simulink model "SMC"  (R2022a)
settings: Solver=ode4  StartTime=0.0  StopTime=30  FixedStep=0.0002  RelTol=1e-3  EnableMultiTasking=on
InitFcn:
  | clc
  | clear
  | x=[    1.0000
  |    -1.0000
  |    -1.0000
  |    -1.0000
  |     1.0000
  |     1.0000
  |     1.0000
  |    -1.0000
  |    -1.0000
  |    -0.0461
  |    -0.2275
  |    -1.0000
  |     1.0000
  |     1.0000
  |     1.0000
  |     1.0000
  |     0.1336
  |    -0.0153
  |    -0.9258
  |     1.0000
  |     1.0000
  |     1.0000
  |    -1.0000
  |     1.0000
  |    -1.0000
  |     1.0000];
  | 
  | x=x';
  | 
  | alpha = 20+5*x(1);
  | beta = 4+2*x(2);
  | 
  | gamma2 = 1.2 + 0.3* x(3);
  | gamma1 = 1.2 + 0.3* x(4);
  | 
  | eta1 = 2.5 + 0.5*x(5);
  | eta2 = 0.3 + 0.1*x(6);
  | 
  | 
  | w1 =25* x(7:15);
  | w4 =abs(5* x(16:24));
  | b1 = 2 + x(25);
  | b4 = 2 + x(26);
  | 
  | 
  | center1=[-0.5 0 0.5];
  | center2=[-2 0 2];
  | 
  | sigma1 = [0.2 0.2 0.2];
  | sigma2 = [0.6 0.6 0.6];
  | 
  | x1=[     1.0000
  |    -0.7700
  |    -0.9968
  |    -0.7959
  |    -0.3103
  |    -0.2531
  |     0.7496
  |     0.6290
  |    -0.6185
  |    -0.2913
  |     0.0215
  |    -0.1400
  |     0.0582
  |     0.8560
  |     0.2296
  |    -0.4623
  |     0.4590
  |    -0.3154
  |     0.7435
  |     0.3255
  |     0.1149
  |    -0.2814
  |    -0.4088
  |     0.2365
  |    -0.7489
  |    -0.0827];
  | 
  | alpha_1 = 22+6*x1(1);
  | beta_1 =5+2*x1(2);
  | 
  | gamma2_1 = 1.2 + 0.4* x1(3);
  | gamma1_1 = 1.2 + 0.4* x1(4);
  | 
  | eta1_1 = 2.5 + 0.5*x1(5);
  | eta2_1 = 0.3 + 0.1*x1(6);
  | 
  | S = 0;
  | 
  | w1_1 =30* x1(7:15) + 5;
  | w4_1 =abs(5* x1(16:24));
StopFcn:
  | save('SMC.mat')
settings Model: Creator=Ali.Assareh  LastModifiedBy=MohammadAli
settings SolverCC: AlgebraicLoopSolver=TrustRegion
settings DataIOCC: LimitDataPoints=on  SaveFormat=Array  ReturnWorkspaceOutputs=off
settings OptimizationCC: LifeSpan=inf
settings DebuggingCC: UnderspecifiedInitializationDetection=Classic  MergeDetectMultiDrivingBlocksExec=none  SolverPrmCheckMsg=warning  UnconnectedInputMsg=warning  UnconnectedOutputMsg=warning  UnconnectedLineMsg=warning  StateNameClashWarn=warning  SFUnexpectedBacktrackingDiag=warning  SFNoUnconditionalDefaultTransitionDiag=warning  SFExecutionAtInitializationDiag=none  SFMachineParentedDataDiag=warning  ArithmeticOperatorsInVariantConditions=warning
settings HardwareCC: ProdBitPerPointer=32  ProdBitPerSizeT=32  ProdBitPerPtrDiffT=32  ProdLargestAtomicFloat=None  ProdIntDivRoundTo=Undefined  ProdEndianess=Unspecified  ProdWordSize=32  ProdHWDeviceType=32-bit Generic
settings ModelReferenceCC: PropagateSignalLabelsOutOfModel=off
settings SFSimCC: SimUseLocalCustomCode=off  CustomCodeUndefinedFunction=UseInterfaceOnly
settings RTWCC: RTWUseLocalCustomCode=off  DLArmComputeVersion=19.05
settings CodeAppCC: StateflowObjectComments=on
settings GRTTargetCC: TargetLangStandard=C89/C90 (ANSI)
settings ConfigComp: CovMetricSettings=dw  CovSaveCumulativeToWorkspaceVar=on  CovSaveSingleToWorkspaceVar=on  CovExternalEMLEnable=off

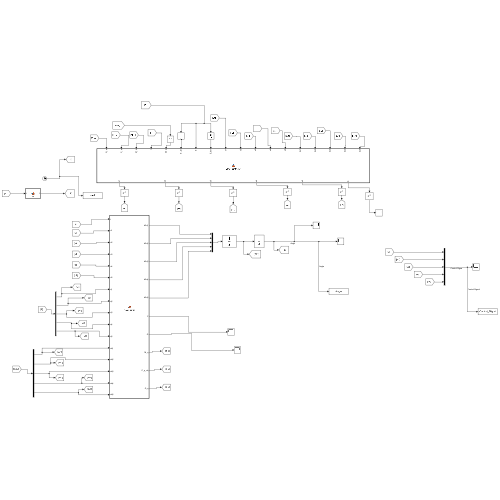
[thumbnail: Simulink's stored preview of the top-level diagram]
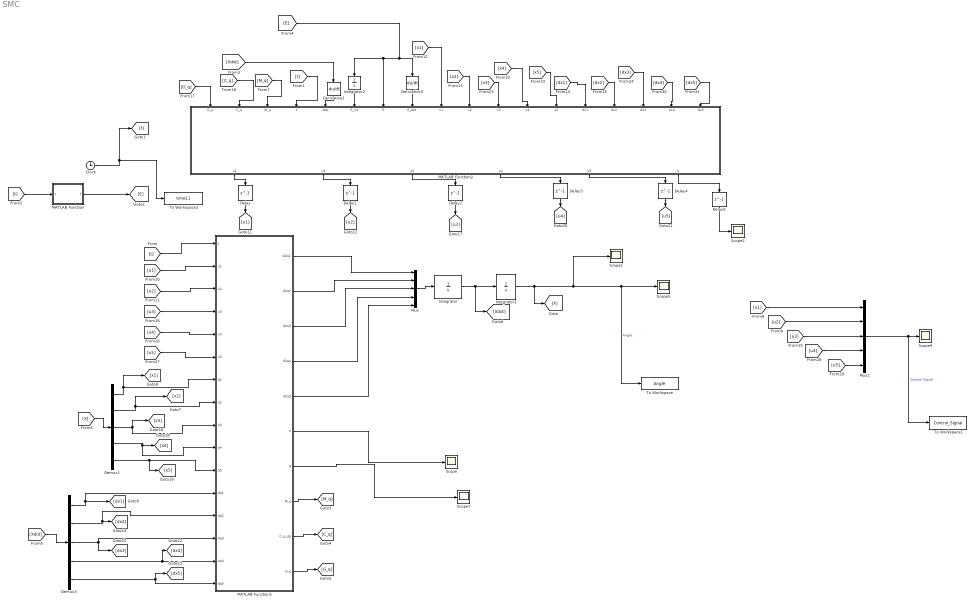
== system SMC ==
  Clock : Clock
  Delay{,1..4,6} (6 alike) : Delay  DelayLength=1  InitialCondition=0
  Demux1 : Demux  Outputs=5
  Demux3 : Demux  Outputs=5
  Derivative1 : Derivative
  Derivative3 : Derivative
  Integrator : Integrator  InitialCondition=[0.4;-0.8;1;0.3;0.1]*1
  Integrator1 : Integrator  InitialCondition=[-0.4;0.8;0.4;-1.7;1.1]*1
  Integrator2 : Integrator
  MATLAB Function : MATLAB Function  TreatAsAtomicUnit=on
  MATLAB Function1 : MATLAB Function  TreatAsAtomicUnit=on
  MATLAB Function2 : MATLAB Function  TreatAsAtomicUnit=on
  Mux : Mux  Inputs=5
  Mux1 : Mux  Inputs=5
  Scope{,1..2,5,7,9} (6 alike) : Scope
  To Workspace : ToWorkspace  VariableName=Angle  SampleTime=-1
  To Workspace1 : ToWorkspace  VariableName=Control_Signal  SampleTime=-1
  To Workspace2 : ToWorkspace  VariableName=time11  SampleTime=-1
  wires:
  MATLAB Function1/1(d2q1) -> Mux/1
  MATLAB Function1/2(d2q2) -> Mux/2
  Integrator/1 -> [Xdot], Integrator1/1
  Mux/1 -> Integrator/1
  Demux3/2 -> MATLAB Function1/13(dq2), [dx2]
  Demux3/1 -> MATLAB Function1/12(dq1), [dx1]
  Clock/1 -> [t], To Workspace2/1
  MATLAB Function2/2(u2) -> Delay1/1
  [t] -> MATLAB Function1/1(t)
  [t] -> MATLAB Function2/4(t)
  [Xdot] -> Demux3/1
  [X] -> Demux1/1
  [E] -> MATLAB Function2/7(E), Integrator2/1, Derivative3/1
  Demux1/1 -> [x1], MATLAB Function1/7(q1)
  Demux1/2 -> MATLAB Function1/8(q2), [x2]
  MATLAB Function2/1(u1) -> Delay/1
  [u1] -> MATLAB Function1/2(u1)
  [u2] -> MATLAB Function1/3(u2)
  MATLAB Function1/7(G) -> Scope7/1
  MATLAB Function1/6(F) -> Scope/1
  Derivative3/1 -> MATLAB Function2/8(E_dot)
  [x1] -> MATLAB Function2/9(x1)
  [x2] -> MATLAB Function2/10(x2)
  [u1] -> Mux1/1
  [u2] -> Mux1/2
  MATLAB Function1/3(d2q3) -> Mux/3
  [u3] -> MATLAB Function1/4(u3)
  Demux3/3 -> MATLAB Function1/14(dq3), [dx3]
  Demux1/3 -> [x3], MATLAB Function1/9(q3)
  MATLAB Function2/3(u3) -> Delay2/1
  [u3] -> Mux1/3
  [x3] -> MATLAB Function2/11(x3)
  [dx3] -> MATLAB Function2/16(dx3)
  MATLAB Function1/4(d2q4) -> Mux/4
  MATLAB Function1/5(d2q5) -> Mux/5
  [u4] -> MATLAB Function1/5(u4)
  [u5] -> MATLAB Function1/6(u5)
  Demux1/4 -> MATLAB Function1/10(q4), [x4]
  Demux1/5 -> MATLAB Function1/11(q5), [x5]
  MATLAB Function2/5(u5) -> Delay4/1
  MATLAB Function2/4(u4) -> Delay3/1
  [u4] -> Mux1/4
  [u5] -> Mux1/5
  Demux3/4 -> [dx4], MATLAB Function1/15(dq4)
  Demux3/5 -> [dx5], MATLAB Function1/16(dq5)
  [dx5] -> MATLAB Function2/18(dx5)
  [x4] -> MATLAB Function2/12(x4)
  [x5] -> MATLAB Function2/13(x5)
  [dx1] -> MATLAB Function2/14(dx1)
  [dx2] -> MATLAB Function2/15(dx2)
  [dx4] -> MATLAB Function2/17(dx4)
  [t] -> MATLAB Function/1(t)
  MATLAB Function/1(f) -> [E]
  Integrator2/1 -> MATLAB Function2/6(E_int)
  [Xdot] -> Derivative1/1
  Derivative1/1 -> MATLAB Function2/5(ddq)
  MATLAB Function1/8(M_q) -> [M_q]
  MATLAB Function1/9(C_q_dq) -> [C_q]
  MATLAB Function1/10(G_q) -> [G_q]
  [M_q] -> MATLAB Function2/3(M_q)
  [C_q] -> MATLAB Function2/2(C_q)
  [G_q] -> MATLAB Function2/1(G_q)
  Delay/1 -> [u1]
  Delay1/1 -> [u2]
  Delay2/1 -> [u3]
  Delay3/1 -> [u4]
  Delay4/1 -> [u5]
  Integrator1/1 -> Scope1/1, To Workspace/1, Scope5/1, [X]  "Angle"
  Mux1/1 -> To Workspace1/1, Scope9/1  "Control Signal"
  MATLAB Function2/6(S) -> Delay6/1
  Delay6/1 -> Scope2/1

== matlab function SMC/MATLAB Function1 ==
  data: t input; u1 input; d2q1 output; u2 input; u3 input; u4 input; u5 input; q1 input; q2 input; q3 input; q4 input; q5 input; dq1 input; dq2 input; d2q2 output; d2q3 output; d2q4 output; d2q5 output; F output; G output; dq3 input; dq4 input; dq5 input; M_q output; C_q_dq output; G_q output
function [d2q1,d2q2,d2q3,d2q4,d2q5,F,G, M_q,C_q_dq,G_q] = manipulator(t,u1,u2,u3,u4,u5,q1,q2,q3,q4,q5,dq1,dq2,dq3,dq4,dq5)

%% initial param

I1 = 1.14;
I2 = 1.43;
I3 = 1.38;
I4 = 0.298;
I5 = -0.0213;
I6 = -0.0142;
I7 = -0.0001;
I8 = 0.372;
I9 = -0.011;
I10 = 0.00125;
I11 = -0.0124;
I12 = 0.000058;
I13 = -0.69;
I14 = 0.134;
I15 = 0.238;
I16 = 0.00379;
I17 = 0.000642;
I18 = 4.71;
I19 = 1.75;
I20 = 0.333;
I21 = 0.000642;
I22 = 0.2;
I23 = 0.00164;
I24 = 0.179;

dq = [dq1,dq2,dq3,dq4,dq5]';
%% calculate M(q)

m11=I2 + I19+I3*cos(q2)^2+I4*sin(q2+q3) + I5*sin(q2+q3)*cos(q2+q3)+I6*sin(q2)*cos(q2)...
    +I7*sin(q2+q3)^2 + 2 +I8*cos(q2)*sin(q2+q3) + I9*cos(q2)*cos(q2+q3)+I10*sin(q2+q3)^2 + ...
    I11 * cos(q2)*sin(q2+q3) + I12*sin(q2+q3)*cos(q2+q3);

m12=I13*sin(q2)+I14*cos(q2+q3)+I12*cos(q2) + I16*sin(q2+q3)-I17*cos(q2+q3);
m21=m12;

m13 = I14*cos(q2+q3) + I16*sin(q2+q3) - I17*cos(q2+q3);
m31=m13;

m22 = I18+I19+I20 + 2*I8*sin(q3)+I9*cos(q2)+I10 + I11*sin(q3);

m23 = I8*sin(q3)+ I20 +I9*cos(q3) + I11*sin(q3) + 2*I10;
m32 =m23;

m33 = I20 + 2*I10;
m35 = I10 + I21;
m53 = m35;
m44 = I22 + I23;
m55 = I24 + I21;

M_q=[m11,m12,m13,0,0
    m21,m22,m23,0,0
    m31,m32,m33,0,m35
    0,0,0,m44,0
    0,0,m53,0,m55];

%% Coriolis/Centrifugal torques matrix

c1 = 2*(-I3*sin(q2)*cos(q2) + I8*cos(2*q2+q3)+ I4*sin(q2+q3)*cos(q2)-I9*sin(2*q2+q3)+...
        -2*I10*sin(q2+q3)+ I11*cos(2*q2+q3) + I7*sin(q2+q3)*cos(q2*q3)+ ...
        I12*(1-2*sin(q2+q3)^2))  +  I5*(1-2*sin(q2+q3)+I6*(1-2*sin(q2)^2));
    
c2 = 2*(-I14*sin(q2+q3)+I16*cos(q2+q3)+I17*sin(q2+q3));

c3 = I13*cos(q2)-I14*sin(q2+q3)-I15*sin(q2)+I16*cos(q2+q3)+I17*sin(q2+q3);

c4 = 2* (I8*cos(q2)*cos(q2+q3)+I4*sin(q2+q3)*cos(q2+q3)-I9*cos(q2)*sin(2*q2)+...
    2*I10*sin(q2+q3)*cos(q2+q3)+I11*cos(q2)*cos(q2+q3)+I7*sin(q2+q3)*cos(q2+q3)+...
    I12*(1-2*sin(q2+q3)))+I5*(1-2*sin(q2+q3));
c5 = 0.5*c2;
c6 =-0.5*c1;
c7 = 2*(-2*I9*sin(q3)+I8*cos(q3)+I11*cos(q3));

c8 = -0.5*c4;
c9 = (1-2*I10)*sin(q2+q3)*cos(q2+q3)-I11*cos(q2)*cos(q2+q3)-I12*cos(q2+q3)^2;
c10 = (-I23+I19+I20)*sin(q2+q3);
c11 = (-I20+I23+I19)*sin(q2+q3);
c12 = -I11*cos(q3)-I12;
    
    
C_q_dq=[c1*dq2 , c2*dq3+c3*dq2, c4*dq2+c5*dq3, 0 , 0
        c6*dq1 , c7*dq3,        c8*dq3,        0 , 0
        c5*dq1 , c9*dq2,        0,             0 , 0
        c10*dq2, 0,             c11*dq1,       0 , 0
        0 ,      c12*dq2,       0,             0 , 0];

%% Gravity Matrix

g1 = -37.2;
g2 = -8.43;
g3 = 1.02;
g4 = 0.249;
g5 = -0.0292;

g2_q= g1*cos(q2) + g3*sin(q2)+ g4*cos(q2+q3)+(g2+g5)*sin(q2+q3);
g3_q= (g2+g5)*sin(q2+q3) + g4*cos(q2+q3);
g5_q= g5*sin(q2+q3);

G_q=[0,g2_q,g3_q,0,g5_q]';


%% disturbance 


f = zeros(5,1);
%% q=[q1,q2,q3,q4,q5]'; output system

u = [u1,u2,u3,u4,u5]';

F = inv(M_q)*(-f-(C_q_dq)*(dq)-(G_q));
G = inv(M_q);
d2q = F + G*u;


d2q1=d2q(1);
d2q2=d2q(2);
d2q3=d2q(3);
d2q4=d2q(4);
d2q5=d2q(5);

== matlab function SMC/MATLAB Function ==
  data: t input; f output
function f = fcn(t)



f=[sin(t-2)
    1.2*cos(t-5)
    1.6*cos(t)
    -1.5*cos(t-5)
    0.7];

== matlab function SMC/MATLAB Function2 ==
  data: G_q input; C_q input; M_q input; t input; ddq input; E_int input; E input; E_dot input; u1 output; x1 input; x2 input; x3 input; x4 input; x5 input; dx1 input; dx2 input; u2 output; u3 output; u4 output; u5 output; dx3 input; dx4 input; dx5 input; S output
function [u1,u2,u3,u4,u5,S]= SMC_controller( G_q, C_q, M_q, t,ddq, E_int, E,E_dot,x1,x2,x3,x4,x5, dx1,dx2,dx3,dx4,dx5)

%% initial parameters

q1 = x1;
q2 = x2;
q3 = x3;
q4 = x4;
q5 = x5;

dq1 = dx1;
dq2 = dx2;
dq3 = dx3;
dq4 = dx4;
dq5 = dx5;

dq = [dq1,dq2,dq3,dq4,dq5]';
q = [q1,q2,q3,q4,q5]';


%% Controller 

K=20;
landa1 = 1;
landa2 = 1;

S = -landa1*E;
S_dot = -landa2*E_dot;

%% u; Signal Control

u  =  - K*dq  - E - 1.5*S_dot;


u1=u(1);
u2=u(2);
u3=u(3);
u4=u(4);
u5=u(5);
